simulink model "TS04_basic_example"  (R2022a)
settings: Solver=ode45  StartTime=0.0  StopTime=180  RelTol=1e-3  EnableMultiTasking=on
undefined symbols (not defined in the file or in its folder): Advantech, PCI
libraries: sldrtlib x4
settings Model: Creator=Admin  LastModifiedBy=admin
settings SolverCC: AlgebraicLoopSolver=TrustRegion
settings DataIOCC: LimitDataPoints=on  SaveFormat=Array  ReturnWorkspaceOutputs=off
settings OptimizationCC: LifeSpan=inf
settings DebuggingCC: UnconnectedInputMsg=warning  UnconnectedOutputMsg=warning  UnconnectedLineMsg=warning  SFUnexpectedBacktrackingDiag=warning  SFNoUnconditionalDefaultTransitionDiag=warning  SFExecutionAtInitializationDiag=none  SFMachineParentedDataDiag=warning  ArithmeticOperatorsInVariantConditions=warning
settings HardwareCC: ProdBitPerPointer=32  ProdBitPerSizeT=32  ProdBitPerPtrDiffT=32  ProdLargestAtomicFloat=None  ProdIntDivRoundTo=Undefined  ProdEndianess=Unspecified  ProdWordSize=32  ProdHWDeviceType=32-bit Generic
settings ModelReferenceCC: EnableRefExpFcnMdlSchedulingChecks=off  PropagateSignalLabelsOutOfModel=off
settings SFSimCC: SimUseLocalCustomCode=off  CustomCodeUndefinedFunction=UseInterfaceOnly
settings RTWCC: RTWUseLocalCustomCode=off
settings CodeAppCC: StateflowObjectComments=on
settings GRTTargetCC: TargetLangStandard=C89/C90 (ANSI)
settings ConfigComp: CovMetricSettings=dw  CovSaveCumulativeToWorkspaceVar=on  CovSaveSingleToWorkspaceVar=on  CovExternalEMLEnable=off

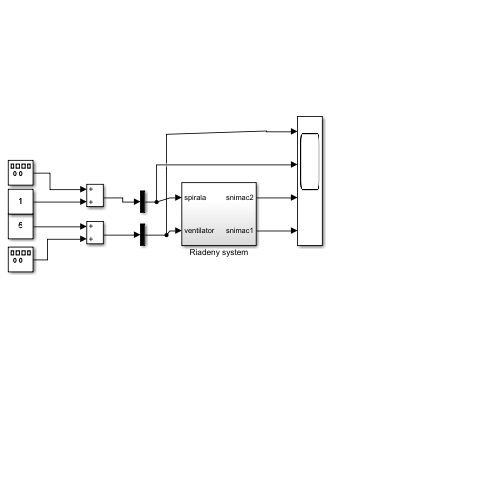
[thumbnail: Simulink's stored preview of the top-level diagram]
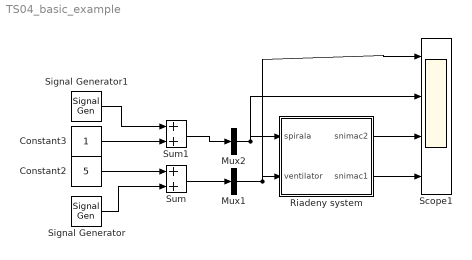
== system TS04_basic_example ==
  Constant2 : Constant  Value=5
  Constant3 : Constant
  Mux1 : Mux  Inputs=1
  Mux2 : Mux  Inputs=1
  Riadeny system : Subsystem
  Scope1 : Scope  NumInputPorts=4
  Signal Generator : SignalGenerator  Amplitude=2  Frequency=0.1
  Signal Generator1 : SignalGenerator  WaveForm=square  Frequency=1/120
  Sum : Sum
  Sum1 : Sum
  wires:
  Mux2/1 -> Scope1/2, Riadeny system/1(spirala)
  Riadeny system/1(snimac2) -> Scope1/3
  Riadeny system/2(snimac1) -> Scope1/4
  Mux1/1 -> Scope1/1, Riadeny system/2(ventilator)
  Signal Generator1/1 -> Sum1/1
  Constant3/1 -> Sum1/2
  Signal Generator/1 -> Sum/2
  Constant2/1 -> Sum/1
  Sum/1 -> Mux1/1
  Sum1/1 -> Mux2/1

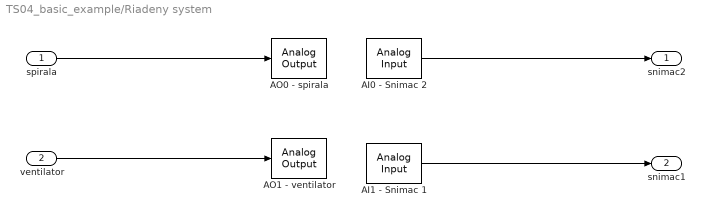
== system TS04_basic_example/Riadeny system ==
  spirala : Inport
  ventilator : Inport  Port=2
  AI0 - Snimac 2 : sldrtlib/Analog Input  SampleTime=0.1  MaxMissedTicks=10  ShowMissedTicks=off  YieldWhenWaiting=off  DrvName=Advantech/PCI-1716  DrvAddress=4294967295  DrvOptions=0  Channels=1  RangeMode=1  VoltRange=1  DataType=1
      settings: AttributesFormatString=Advantech\nPCI-1716 [auto]
  AI1 - Snimac 1 : sldrtlib/Analog Input  SampleTime=0.1  MaxMissedTicks=10  ShowMissedTicks=off  YieldWhenWaiting=off  DrvName=Advantech/PCI-1716  DrvAddress=4294967295  DrvOptions=0  Channels=2  RangeMode=1  VoltRange=1  DataType=1
      settings: AttributesFormatString=Advantech\nPCI-1716 [auto]
  AO0 - spirala : sldrtlib/Analog Output  SampleTime=0.1  MaxMissedTicks=10  ShowMissedTicks=off  YieldWhenWaiting=off  DrvName=Advantech/PCI-1716  DrvAddress=4294967295  DrvOptions=0  Channels=1  RangeMode=1  VoltRange=4  InitialValue=[]  FinalValue=[]
      settings: AttributesFormatString=Advantech\nPCI-1716 [auto]
  AO1 - ventilator : sldrtlib/Analog Output  SampleTime=0.1  MaxMissedTicks=10  ShowMissedTicks=off  YieldWhenWaiting=off  DrvName=Advantech/PCI-1716  DrvAddress=4294967295  DrvOptions=0  Channels=2  RangeMode=1  VoltRange=4  InitialValue=[]  FinalValue=[]
      settings: AttributesFormatString=Advantech\nPCI-1716 [auto]
  snimac2 : Outport
  snimac1 : Outport  Port=2
  wires:
  spirala/1 -> AO0 - spirala/1
  ventilator/1 -> AO1 - ventilator/1
  AI0 - Snimac 2/1 -> snimac2/1
  AI1 - Snimac 1/1 -> snimac1/1
